simulink model "MultirotorPx4PitchOnly"  (R2018b)
settings: Solver=VariableStepAuto  StartTime=0.0  StopTime=100  RelTol=1e-3
undefined symbols (not defined in the file): Ctrl, Uav
libraries: simulink_extras x2, QuaternionLibrary x1
settings Model: Creator=jban039  LastModifiedBy=jeremie
settings OptimizationCC: AccelVerboseBuild=on

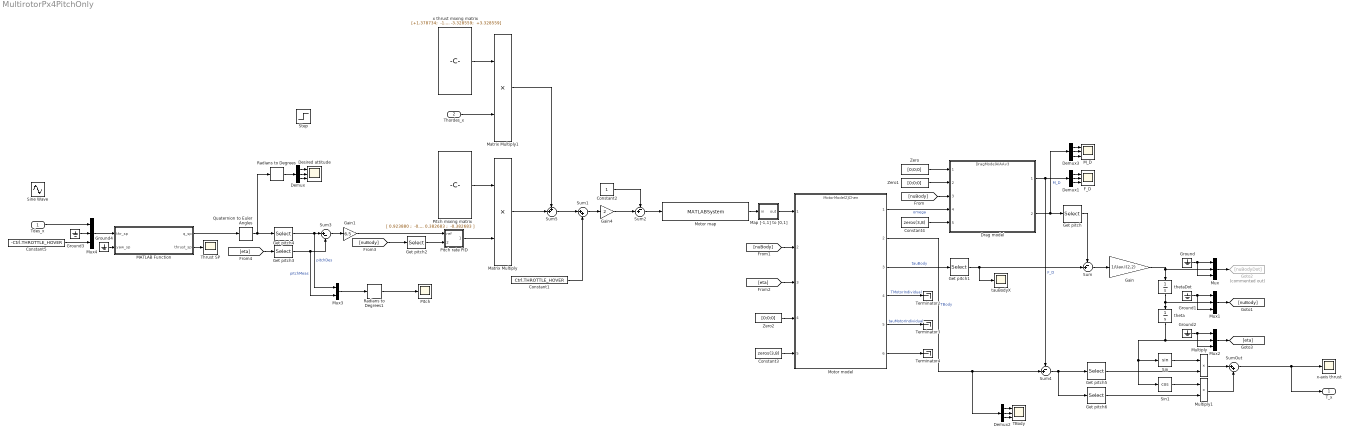
== system MultirotorPx4PitchOnly ==
  Tdes_x : Inport
  Thordes_x : Inport  Port=2
  Constant1 : Constant  Value=Ctrl.THROTTLE_HOVER
  Constant2 : Constant
  Constant3 : Constant  Value=zeros(3,8)
  Constant4 : Constant  Value=zeros(3,8)
  Constant5 : Constant  Value=-Ctrl.THROTTLE_HOVER
  Demux{,1..3} (4 alike) : Demux  Outputs=3
  Desired attitude : Scope  NumInputPorts=3
  Drag model : ModelReference  ModelNameDialog=DragModelAIAAv3  SimulationMode=Normal  ModelReferenceVersion=1.373
  F_D : Scope  NumInputPorts=3
  Gain : Gain  Gain=1/Uav.I(2,2)
  Gain1 : Gain  Gain=6.5
  Gain4 : Gain  Gain=2
  Get pitch{,1..4} (5 alike) : Selector  InputPortWidth=3  IndexOptions=Index vector (dialog)  Indices=[2]  OutputSizes=1
  Get pitch5 : Selector  InputPortWidth=3  IndexOptions=Index vector (dialog)  Indices=[3]  OutputSizes=1
  Get pitch6 : Selector  InputPortWidth=3  IndexOptions=Index vector (dialog)  Indices=[1]  OutputSizes=1
  Goto2 : Goto  Commented=on  GotoTag=nuBodyDot
  Ground{,1..4} (5 alike) : Ground
  MATLAB Function : MATLAB Function  TreatAsAtomicUnit=on
  M_D : Scope  NumInputPorts=3
  Map [-1,1] to [0,1] : Subsystem
  Matrix Multiply : Product
  Matrix Multiply1 : Product
  Motor map : MATLABSystem  System=MotorMap  airframeConfig=5  SimulateUsing=Code generation
      mask Type: MotorMap
      mask Display:
      | disp(['MOTOR' char(10) 'MAP' char(10) 'octa_x']);
      | port_label('input',1,'px4PWM');
      | port_label('output',1,'simPWM');
  Motor model : ModelReference  ModelNameDialog=MotorModelZJChen  SimulationMode=Normal  ModelReferenceVersion=1.444
  Multiply : Product
  Multiply1 : Product
  Mux{,1..2,4} (4 alike) : Mux  Inputs=3
  Mux3 : Mux  Inputs=2
  Pitch : Scope
  Pitch mixing matrix : Constant  Value=|  VectorParams1D=off
      | [ 0.923880 ;
      |  -0.923880 ;
      |   0.382683 ;
      |  -0.923880 ;
      |   0.923880 ;
      |  -0.382683 ;
      |   0.382683 ;
      |  -0.382683 ]
  Pitch rate PID : Subsystem  mask{PID_P=0.15, PID_I=0.05, PID_D=0.003, PID_FC=30, PID_I_STATENAME='AttRatePID_I_pitch', PID_D_STATENAME='AttRatePID_D_pitch'}
      mask prompts: PID_P "P gain"; PID_I "I gain"; PID_D "D gain"; PID_FC "D filter cutoff (Hz)"; PID_I_STATENAME "Integartor state name"; PID_D_STATENAME "D filter state name"
      mask DialogControl DescGroupVar Prompt: PID Controller with Second Order Derivative Filter
      mask DialogControl DescTextVar Prompt: The derivative gain is applied on the derivative of y rather than that of the error (r-y).
      mask Display:
      | disp('PID(s)')
      | port_label('input', 1, 'r')
      | port_label('input', 2, 'y')
      | text(1,0,'2^{nd}','horizontalAlignment','right','interpreter','tex','verticalAlignment','bottom')
  Quaternion to Euler Angles : QuaternionLibrary/Quaternion to Euler Angles
  Radians to Degrees : simulink_extras/Transformations/Radians to Degrees
  Radians to Degrees1 : simulink_extras/Transformations/Radians to Degrees
  Sin : Trigonometry
  Sin1 : Trigonometry  Operator=cos
  Sine Wave : Sin  Amplitude=0.1  Frequency=30  SampleTime=0
  Step : Step  After=0.1  SampleTime=0
  Sum : Sum  Inputs=-+|
  Sum1 : Sum  Inputs=|++
  Sum2 : Sum  Inputs=-+|
  Sum3 : Sum  Inputs=|+-
  Sum4 : Sum  Inputs=-+|
  Sum5 : Sum  Inputs=++|
  SumOut : Sum  Inputs=|++
  TBody : Scope  NumInputPorts=3
  Terminator2 : Terminator
  Terminator3 : Terminator
  Terminator4 : Terminator
  Thrust SP : Scope
  Zero : Constant  Value=[0;0;0]  OutDataTypeStr=Inherit: Inherit via back propagation
  Zero1 : Constant  Value=[0;0;0]  OutDataTypeStr=Inherit: Inherit via back propagation
  Zero2 : Constant  Value=[0;0;0]  OutDataTypeStr=Inherit: Inherit via back propagation
  tauBodyX : Scope
  theta : Integrator
  thetaDot : Integrator  ContinuousStateAttributes='thetaDDot'
  x thrust mixing matrix : Constant  Value=|  VectorParams1D=off
      | [+1.378734;
      |  -1.378734;
      |  -3.328559;
      |  -1.378734;
      |  +1.378734;
      |  +3.328559;
      |  -3.328559;
      |  +3.328559]
  x-axis thrust : Scope
  T_x : Outport
  wires:
  Pitch rate PID/1(Out) -> Matrix Multiply/2
  Pitch mixing matrix/1 -> Matrix Multiply/1
  Constant2/1 -> Sum2/1
  Gain4/1 -> Sum2/2
  Matrix Multiply/1 -> Sum5/2
  Map [-1,1] to [0,1]/1(out) -> Motor model/1
  Motor map/1 -> Map [-1,1] to [0,1]/1(in)
  Sum2/1 -> Motor map/1
  Sum1/1 -> Gain4/1
  Constant1/1 -> Sum1/2
  Motor model/1 -> Drag model/4  "omega"
  Drag model/1 -> Sum4/1, Demux1/1  "F_D"
  Get pitch1/1 -> tauBodyX/1, Sum/2
  Get pitch/1 -> Sum/1
  Sum/1 -> Gain/1
  Gain/1 -> thetaDot/1, Mux/2
  Zero/1 -> Drag model/1
  Zero1/1 -> Drag model/2
  Zero2/1 -> Motor model/4
  Constant3/1 -> Motor model/5
  Ground/1 -> Mux/3, Mux/1
  Ground1/1 -> Mux1/1, Mux1/3
  thetaDot/1 -> Mux1/2, theta/1
  Ground2/1 -> Mux2/3, Mux2/1
  Mux1/1 -> [nuBody]
  Mux/1 -> Goto2/1
  Motor model/3 -> Get pitch1/1  "tauBody"
  Mux2/1 -> [eta]
  [nuBody] -> Drag model/3
  Constant4/1 -> Drag model/5
  [nuBody] -> Motor model/2
  [eta] -> Motor model/3
  Motor model/2 -> Demux2/1, Sum4/2  "TBody"
  Gain1/1 -> Pitch rate PID/1(ref)
  Motor model/4 -> Terminator2/1  "TMotorIndividual"
  Motor model/5 -> Terminator3/1  "tauMotorIndividual"
  Motor model/6 -> Terminator4/1
  [nuBody] -> Get pitch2/1
  Sum3/1 -> Gain1/1
  [eta] -> Get pitch3/1
  Get pitch4/1 -> Mux3/1, Sum3/1  "pitchDes"
  Mux3/1 -> Radians to Degrees1/1
  Get pitch2/1 -> Pitch rate PID/2(meas)
  Get pitch3/1 -> Mux3/2, Sum3/2  "pitchMeas"
  MATLAB Function/1(q_sp) -> Quaternion to Euler Angles/1
  Mux4/1 -> MATLAB Function/1(thr_sp)
  Constant5/1 -> Mux4/3
  Tdes_x/1 -> Mux4/1
  Ground3/1 -> Mux4/2
  MATLAB Function/2(thrust_sp) -> Thrust SP/1
  Quaternion to Euler Angles/1 -> Get pitch4/1, Radians to Degrees/1
  Demux/1 -> Desired attitude/1
  Demux/2 -> Desired attitude/2
  Demux/3 -> Desired attitude/3
  Radians to Degrees/1 -> Demux/1
  theta/1 -> Mux2/2, Sin1/1, Sin/1
  Sin/1 -> Multiply/1
  Get pitch5/1 -> Multiply/2
  SumOut/1 -> T_x/1, x-axis thrust/1
  Sum4/1 -> Get pitch6/1, Get pitch5/1
  Ground4/1 -> MATLAB Function/2(yaw_sp)
  Demux1/3 -> F_D/3
  Demux1/2 -> F_D/2
  Demux1/1 -> F_D/1
  Demux2/1 -> TBody/1
  Demux2/2 -> TBody/2
  Demux2/3 -> TBody/3
  Demux3/1 -> M_D/1
  Demux3/2 -> M_D/2
  Demux3/3 -> M_D/3
  Drag model/2 -> Demux3/1, Get pitch/1  "M_D"
  x thrust mixing matrix/1 -> Matrix Multiply1/1
  Thordes_x/1 -> Matrix Multiply1/2
  Sum5/1 -> Sum1/1
  Matrix Multiply1/1 -> Sum5/1
  Radians to Degrees1/1 -> Pitch/1
  Get pitch6/1 -> Multiply1/2
  Sin1/1 -> Multiply1/1
  Multiply/1 -> SumOut/1
  Multiply1/1 -> SumOut/2

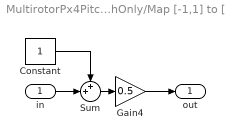
== system MultirotorPx4PitchOnly/Map [-1,1] to [0,1] ==
  in : Inport
  Constant : Constant
  Gain4 : Gain  Gain=0.5
  Sum : Sum  Inputs=++|
  out : Outport
  wires:
  Constant/1 -> Sum/1
  in/1 -> Sum/2
  Gain4/1 -> out/1
  Sum/1 -> Gain4/1

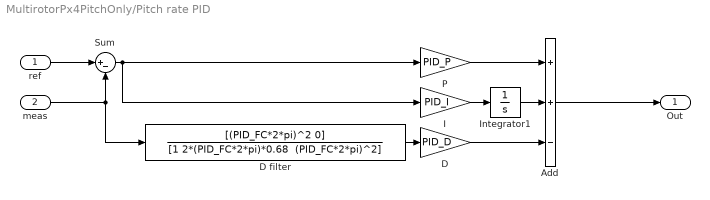
== system MultirotorPx4PitchOnly/Pitch rate PID ==
  ref : Inport
  meas : Inport  Port=2
  Add : Sum  Inputs=++-
  D : Gain  Gain=PID_D
  D filter : TransferFcn  Numerator=[(PID_FC*2*pi)^2 0]  Denominator="[1 2*(PID_FC*2*pi)*0.68  (PID_FC*2*pi)^2]"  ContinuousStateAttributes=PID_D_STATENAME
  I : Gain  Gain=PID_I
  Integrator1 : Integrator  LimitOutput=on  UpperSaturationLimit=0.3  LowerSaturationLimit=-0.3  ContinuousStateAttributes=PID_I_STATENAME
  P : Gain  Gain=PID_P
  Sum : Sum  Inputs=|+-
  Out : Outport
  wires:
  meas/1 -> Sum/2, D filter/1
  ref/1 -> Sum/1
  I/1 -> Integrator1/1
  D/1 -> Add/3
  Sum/1 -> I/1, P/1
  D filter/1 -> D/1
  Integrator1/1 -> Add/2
  P/1 -> Add/1
  Add/1 -> Out/1

== matlab function MultirotorPx4PitchOnly/MATLAB Function ==
  data: thr_sp input size=3; q_sp output; yaw_sp input; thrust_sp output
function [q_sp, thrust_sp] = thrustToAttitude( thr_sp, yaw_sp )

    yaw_body = yaw_sp;
    body_z = -thr_sp./norm(thr_sp);
    
    y_C = [ -sin(yaw_body); cos(yaw_body); 0 ];
    
    body_x = zeros(3,1);
    if body_z(3) > 0.000001
        body_x = cross( y_C, body_z );
        if ( body_z(3) < 0 )
            body_x = -body_x;
        end
        
        body_x = body_x ./ norm(body_x);
    else
        body_x(3) = 1;
    end
    
    body_y = cross( body_z, body_x );
    
    R_sp = [ body_x, body_y, body_z ];
    
    q_sp = from_dcm( R_sp );
    
    thrust_sp = -norm( thr_sp );
    
end

function data  = from_dcm( dcm )
% FROM_DCM Convert DCM to quaternion
% From https://github.com/PX4/Firmware/blob/master/src/lib/mathlib/math/Quaternion.hpp
    data = zeros(4,1);
    tr = dcm(1,1) + dcm(2,2) + dcm(3,3);
    if (tr > 0.0)
        s = sqrt(tr + 1.0);
        data(1) = s * 0.5;
        s = 0.5 / s;
        data(2) = (dcm(3,2) - dcm(2,3) ) * s;
        data(3) = (dcm(1,3) - dcm(3,1) ) * s;
        data(4) = (dcm(2,1) - dcm(1,2) ) * s;
    else
        % Find maximum diagonal element in dcm
        % store index in dcm_i
        dcm_i = 1;
        for i = 2:3 % (int i = 1; i < 3; i++)
            if ( dcm(i,i) > dcm(dcm_i,dcm_i) )
                dcm_i = i;
            end
        end
        dcm_j = rem( ( (dcm_i-1) + 1), 3) + 1;
        dcm_k = rem( ( (dcm_i-1) + 2), 3) + 1;
        s = sqrt( (dcm(dcm_i, dcm_i) - dcm(dcm_j, dcm_j) - ...
            dcm(dcm_k,dcm_k)) + 1.0 );
        data(dcm_i + 1) = s * 0.5;
        s = 0.5 / s;
        data(dcm_j + 1) = ( dcm(dcm_i,dcm_j) + dcm(dcm_j,dcm_i) ) * s;
        data(dcm_k + 1) = ( dcm(dcm_k,dcm_i) + dcm(dcm_i,dcm_k) ) * s;
        data(1) = ( dcm(dcm_k,dcm_j) - dcm(dcm_j,dcm_k) ) * s;
    end
end
